simulink model "runMyArm"  (R2021a)
settings: Solver=FixedStepAuto  StartTime=0.0  StopTime=10  FixedStep=0.1  RelTol=1e-3  EnableMultiTasking=on
values from neighbouring files (symbols this model uses):
  qr = [0; 0; 0; 0; 0; 0]    [ScrewFK.m]    (also in ScrewFK_SCARA.m = [0; 0; 0; 20]; ScrewIK.m; ScrewIK1.m = [0 pi/4 0 pi/2 pi/4 0]'; ScrewIK2.m = [pi/2; -pi/3; pi/6; -pi/6; -pi/3; 0])
  s = QuinticTimeScaling(Tf, timegap * (i - 1))    [Cartesian_Trajectory.m]    (also in CircularTimeScaling.m = t / Tf; CircularTrajectory.m = CircularTimeScaling(Tf,timegap * (i - 1)); InverseKin6R.m = sqrt(r^2 + z_P^2); LinearTimeScaling.m = 10 * (t / Tf)^3 - 15 * (t / Tf)^4 + 6 * (t / Tf)^5)
  X = fprintf('Sine theta at the denominator is zero')    [CircularTrajectory.m]
undefined symbols (not defined in the file or in its folder): jointList, trajList, Y, Z
libraries: sm_lib x45, nesl_utility x22, vrlib x1
(part 2 of 2)

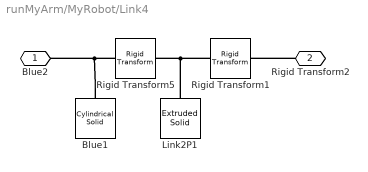
== system runMyArm/MyRobot/Link4 ==
  Blue1 : sm_lib/Body Elements/Cylindrical Solid  GraphicAmbientColor=[0.15 0.15 0.15 1.0]  BasedOnType=Density  CenterOfMass=[0 0 0]  CenterOfMassUnits=m  GraphicDiffuseColor=[0.0 0.0 0.6]  CylinderLength=80  CylinderLengthUnits=cm  CylinderRadius=10  CylinderRadiusUnits=cm  Density=1000  DensityUnits=kg/m^3  DoExposeReferenceFrame=on  GraphicEmissiveColor=[0.0 0.0 0.0 1.0]  ExportEntireGeometry=off  SerializedFrames=<Frames/>  MarkerShape=Sphere  MarkerSize=10  GraphicType=FromGeometry  InertiaType=CalculateFromGeometry  Mass=1  MassUnits=kg  MomentsOfInertia=[1 1 1]  MomentsOfInertiaUnits=kg*m^2  GraphicOpacity=1.0  ProductsOfInertia=[0 0 0]  ProductsOfInertiaUnits=kg*m^2  GraphicShininess=75  GraphicSpecularColor=[0.5 0.5 0.5 1.0]  GraphicVisPropType=SimpleVisualProperties
  Link2P1 : sm_lib/Body Elements/Extruded Solid  GraphicAmbientColor=[0.15 0.15 0.15 1.0]  BasedOnType=Density  CenterOfMass=[0 0 0]  CenterOfMassUnits=m  GraphicDiffuseColor=[0.8 0.4 0.0]  ExportConvexHullGeometry=off  ExtrusionCrossSection=LinkTwo  ExtrusionCrossSectionUnits=cm  Density=1000  DensityUnits=kg/m^3  DoExposeReferenceFrame=on  GraphicEmissiveColor=[0.0 0.0 0.0 1.0]  ExportEntireGeometry=off  ExtrusionLength=35  ExtrusionLengthUnits=cm  ExtrusionType=General  SerializedFrames=<Frames/>  MarkerShape=Sphere  MarkerSize=10  GraphicType=FromGeometry  InertiaType=CalculateFromGeometry  Mass=1  MassUnits=kg  MomentsOfInertia=[1 1 1]  MomentsOfInertiaUnits=kg*m^2  PolygonNumSides=3  GraphicOpacity=1.0  PolygonOuterRadius=1  PolygonOuterRadiusUnits=m  ProductsOfInertia=[0 0 0]  ProductsOfInertiaUnits=kg*m^2  GraphicShininess=75  GraphicSpecularColor=[0.5 0.5 0.5 1.0]  GraphicVisPropType=SimpleVisualProperties
  Rigid Transform1 : sm_lib/Frames and Transforms/Rigid Transform  TranslationMethod=StandardAxis  TranslationStandardOffset=10  TranslationLengthUnit=cm  TranslationStandardAxis=-X  TranslationCartesianOffset=[0 0 0]  TranslationROffset=0  TranslationROffsetUnits=m  TranslationZOffset=0  TranslationZOffsetUnits=m  TranslationThetaOffset=0  TranslationThetaOffsetUnits=deg  RotationMethod=StandardAxis  RotationAngleUnits=deg  RotationStandardAxis=+Y  RotationAngle=180  RotationArbitraryAxis=[0 0 1]  FollAlignAxisA=+X  BaseAlignAxisA=+Y  FollAlignAxisB=+Y  BaseAlignAxisB=+Z  RotationSequenceAxes=FollowerAxes  RotationSequence=XYX  RotationSequenceAngles=[0 0 0]  RotationSequenceAnglesUnits=deg  RotationMatrix=[1 0 0; 0 1 0; 0 0 1]
  Rigid Transform5 : sm_lib/Frames and Transforms/Rigid Transform  TranslationMethod=StandardAxis  TranslationStandardOffset=40  TranslationLengthUnit=cm  TranslationStandardAxis=+Z  TranslationCartesianOffset=[0 0 0]  TranslationROffset=0  TranslationROffsetUnits=m  TranslationZOffset=0  TranslationZOffsetUnits=m  TranslationThetaOffset=0  TranslationThetaOffsetUnits=deg  RotationMethod=StandardAxis  RotationAngleUnits=deg  RotationStandardAxis=+Y  RotationAngle=90  RotationArbitraryAxis=[0 0 1]  FollAlignAxisA=+X  BaseAlignAxisA=+Y  FollAlignAxisB=+Y  BaseAlignAxisB=+Z  RotationSequenceAxes=FollowerAxes  RotationSequence=XYX  RotationSequenceAngles=[0 0 0]  RotationSequenceAnglesUnits=deg  RotationMatrix=[1 0 0; 0 1 0; 0 0 1]
  Blue2 : PMIOPort  Side=Left
  Rigid Transform2 : PMIOPort  Port=2  Side=Right
  connections:
  Rigid Transform1/LConn1 -- Link2P1/RConn1 -- Rigid Transform5/RConn1
  Rigid Transform2/RConn1 -- Rigid Transform1/RConn1
  Rigid Transform5/LConn1 -- Blue2/RConn1 -- Blue1/RConn1

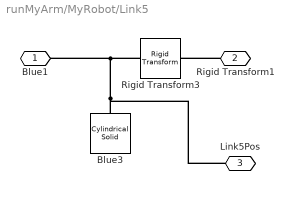
== system runMyArm/MyRobot/Link5 ==
  Blue3 : sm_lib/Body Elements/Cylindrical Solid  GraphicAmbientColor=[0.15 0.15 0.15 1.0]  BasedOnType=Density  CenterOfMass=[0 0 0]  CenterOfMassUnits=m  GraphicDiffuseColor=[0.4 0.8 0.0]  CylinderLength=30  CylinderLengthUnits=cm  CylinderRadius=12  CylinderRadiusUnits=cm  Density=1000  DensityUnits=kg/m^3  DoExposeReferenceFrame=on  GraphicEmissiveColor=[0.0 0.0 0.0 1.0]  ExportEntireGeometry=off  SerializedFrames=<Frames/>  MarkerShape=Sphere  MarkerSize=10  GraphicType=FromGeometry  InertiaType=CalculateFromGeometry  Mass=1  MassUnits=kg  MomentsOfInertia=[1 1 1]  MomentsOfInertiaUnits=kg*m^2  GraphicOpacity=1.0  ProductsOfInertia=[0 0 0]  ProductsOfInertiaUnits=kg*m^2  GraphicShininess=75  GraphicSpecularColor=[0.5 0.5 0.5 1.0]  GraphicVisPropType=SimpleVisualProperties
  Rigid Transform3 : sm_lib/Frames and Transforms/Rigid Transform  TranslationMethod=StandardAxis  TranslationStandardOffset=10  TranslationLengthUnit=cm  TranslationStandardAxis=+X  TranslationCartesianOffset=[0 0 0]  TranslationROffset=0  TranslationROffsetUnits=m  TranslationZOffset=0  TranslationZOffsetUnits=m  TranslationThetaOffset=0  TranslationThetaOffsetUnits=deg  RotationMethod=StandardAxis  RotationAngleUnits=deg  RotationStandardAxis=+Y  RotationAngle=90  RotationArbitraryAxis=[0 0 1]  FollAlignAxisA=+X  BaseAlignAxisA=+Y  FollAlignAxisB=+Y  BaseAlignAxisB=+Z  RotationSequenceAxes=FollowerAxes  RotationSequence=XYX  RotationSequenceAngles=[0 0 0]  RotationSequenceAnglesUnits=deg  RotationMatrix=[1 0 0; 0 1 0; 0 0 1]
  Blue1 : PMIOPort  Side=Left
  Rigid Transform1 : PMIOPort  Port=2  Side=Right
  Link5Pos : PMIOPort  Port=3  Side=Right
  connections:
  Rigid Transform3/LConn1 -- Link5Pos/RConn1 -- Blue3/RConn1 -- Blue1/RConn1
  Rigid Transform1/RConn1 -- Rigid Transform3/RConn1

== stateflow chart runMyArm/Manager1 ==
  state IterateJointAngles
    entry,during:
    jointPos = jointList(:,i)';
  state LoopEachTraj
    entry:
    i = i+1;
  (default) -> IterateJointAngles : {i=1;}
  LoopEachTraj -> IterateJointAngles : [i  <= size(jointList,2)]
  IterateJointAngles -> LoopEachTraj
  data: i local size=1; jointList input; jointPos output size=[1 6]

== stateflow chart runMyArm/Manager ==
  state IterateTrajPoints
    entry,during:
    Pos=saturatePos(trajList(1,i),trajList(2,i),trajList(3,i));
    targetPos = trajList(:,i)';
    targetPos(1,1) = Pos(1,1);
    targetPos(1,2) = Pos(2,1);
    targetPos(1,3) = Pos(3,1);
  state LoopEachTraj
    entry:
    i = i+1;
  state WithinBoundPos = saturatePos(x,y,z) [function]
  (default) -> IterateTrajPoints : {i=1;}
  LoopEachTraj -> IterateTrajPoints : [i  <= size(trajList,2)]
  IterateTrajPoints -> LoopEachTraj
  data: x function_input double size=1; WithinBoundPos function_output; y function_input double size=1; z function_input double size=1; targetPos output size=[1 6]; Pos local size=3; i local size=1; trajList input

== matlab function runMyArm/Manager/saturatePos/each func ==
  data: X input; out output; Y input; Z input
function out = each(X,Y,Z)
if(-260 <= X && X <= 260)
    X = X+0;
elseif(X < -260)
    X = -260;
elseif (X > 260)
    X = 260;
end

if(-260 <= Y && Y <= 260)
    Y = Y+0;
elseif(Y < -260)
    Y = -260;
elseif (Y > 260)
    Y = 260;
end

if(0 <= Z && Z <= 300)
    Z = Z+0;
elseif(Z < 0)
    Z = 0;
elseif (Z > 300)
    Z = 300;
end

out = [X;Y;Z];

end
